simulink model "identification_sl"  (R2021b)
settings: Solver=FixedStepDiscrete  StartTime=0.0  StopTime=inf  FixedStep=0.5  RelTol=1e-3
undefined symbols (not defined in the file): arduino, fclose
libraries: sldrtlib x1
settings Model: Creator=IST  LastModifiedBy=IST

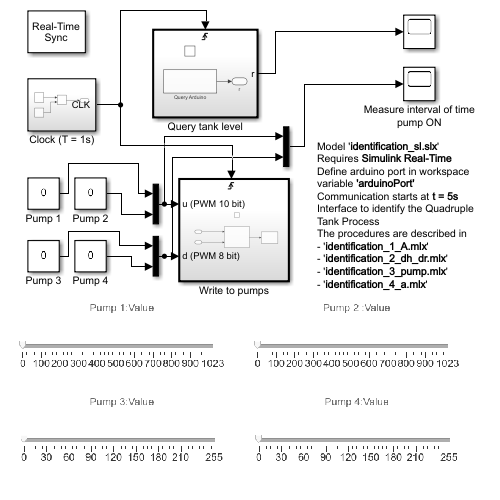
[thumbnail: Simulink's stored preview of the top-level diagram]
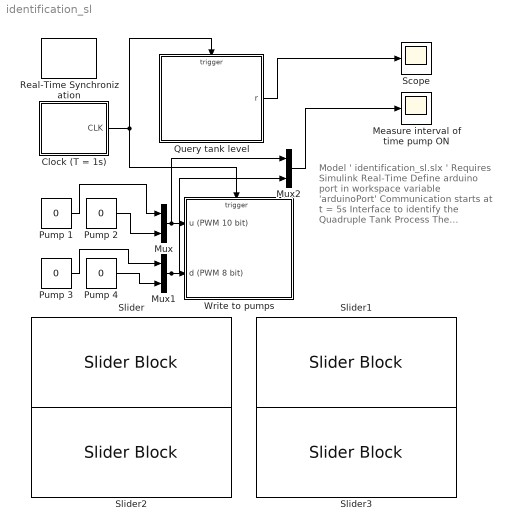
== system identification_sl ==
  note: Model ' identification_sl.slx '
      | Requires Simulink Real-Time
      | Define arduino port in workspace variable 'arduinoPort'
      | Communication starts at t = 5s
      | Interface to identify the Quadruple Tank Process
      | The procedures are described in
      | - ' identification_1_A.mlx '
      | - ' identification_2_dh_dr.mlx '
      | - ' identification_3_pump.mlx '
      | - ' identification_4_a.mlx '
  Clock (T = 1s) : Subsystem
  Measure interval of time pump ON : Scope
  Mux : Mux  Inputs=2
  Mux1 : Mux  Inputs=2
  Mux2 : Mux  Inputs=2
  Pump 1 : Constant  Value=0
  "Pump 2 " : Constant  Value=0
  Pump 3 : Constant  Value=0
  Pump 4 : Constant  Value=0
  Query tank level : Subsystem  Priority=1  InitFcn=|  StopFcn=fclose(arduino)
      | if exist('arduinoPort')
      | if ~isempty(instrfind)
      | fclose(instrfind);
      | delete(instrfind);
      | end
      | arduino = serial(arduinoPort,...
      |                 'BaudRate',9600,...
      |                 'ByteOrder','bigEndian',...
      |                 'DataBits',8,...
      |                 'StopBits',1,...
      |                 'Terminator','');
      | arduino.Parity = 'none';
      | fopen(arduino);
      | else
      | error("Error: Arduino port undefined. Define the port in workspace variable 'arduinoPort'.");
      | end
  Real-Time Synchronization : sldrtlib/Real-Time Synchronization  SampleTime=0.5  MaxMissedTicks=10  ShowMissedTicks=off  YieldWhenWaiting=off
  Scope : Scope
  Slider : SliderBlock  ScaleMax=1023
  Slider1 : SliderBlock  ScaleMax=1023
  Slider2 : SliderBlock  ScaleMax=255
  Slider3 : SliderBlock  ScaleMax=255
  Write to pumps : Subsystem  Priority=2
  wires:
  Mux1/1 -> Mux2/2, Write to pumps/2(d (PWM 8 bit))
  Query tank level/1(r) -> Scope/1
  Mux/1 -> Mux2/1, Write to pumps/1(u (PWM 10 bit))
  Pump 3/1 -> Mux1/1
  Pump 4/1 -> Mux1/2
  Clock (T = 1s)/1("CLK ") -> Write to pumps/Trigger, Query tank level/Trigger
  Pump 1/1 -> Mux/1
  "Pump 2 "/1 -> Mux/2
  Mux2/1 -> Measure interval of time pump ON/1

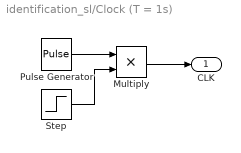
== system identification_sl/Clock (T = 1s) ==
  Multiply : Product
  Pulse Generator : DiscretePulseGenerator  PulseType=Time based  Period=1  PulseWidth=50
  Step : Step  Time=5  SampleTime=0
  "CLK " : Outport  VectorParamsAs1DForOutWhenUnconnected=off
  wires:
  Step/1 -> Multiply/2
  Pulse Generator/1 -> Multiply/1
  Multiply/1 -> "CLK "/1

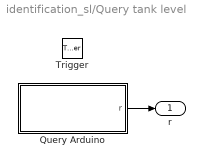
== system identification_sl/Query tank level ==
  Trigger : TriggerPort  VariantControl=Variant  PortDimensions=1
  Query Arduino : MATLAB Function  TreatAsAtomicUnit=on
  r : Outport  VectorParamsAs1DForOutWhenUnconnected=off
  wires:
  Query Arduino/1(r) -> r/1

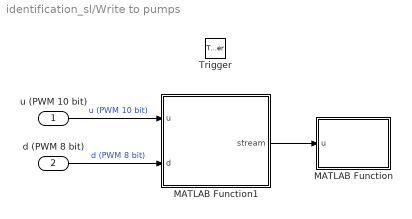
== system identification_sl/Write to pumps ==
  u (PWM 10 bit) : Inport
  d (PWM 8 bit) : Inport  Port=2
  Trigger : TriggerPort  VariantControl=Variant  PortDimensions=1
  MATLAB Function : MATLAB Function  TreatAsAtomicUnit=on
  MATLAB Function1 : MATLAB Function  TreatAsAtomicUnit=on
  wires:
  u (PWM 10 bit)/1 -> MATLAB Function1/1(u)  "u (PWM 10 bit)"
  d (PWM 8 bit)/1 -> MATLAB Function1/2(d)  "d (PWM 8 bit)"
  MATLAB Function1/1(stream) -> MATLAB Function/1(u)

== matlab function identification_sl/Write to pumps/MATLAB Function ==
  data: u input
function toArduino(u)
% Find arduino serial object
coder.extrinsic('instrfind'); 
persistent arduino;
if isempty(arduino)
    arduino = instrfind('Status','open','Baud',9600);
end
% Send metadata
fprintf(arduino, "#16");
% Send actuation inputs
fwrite(arduino,u,'uint16');
end

== matlab function identification_sl/Query tank level/Query Arduino ==
  data: r output
function r = queryArduino()
% Find arduino serial object
coder.extrinsic('instrfind'); 
persistent arduino;
if isempty(arduino)
    arduino = instrfind('Status','open','Baud',9600);
end

% Query arduino
fprintf(arduino, '$');
% Ignore metadata
fread(arduino,[4 1],'uint8');
% Read water-level data
aux = fread(arduino,[5 1],'uint16');
u = zeros(5,1);
u(5) = double(aux(5,1));
for i = 1:4
    u(i) = double(aux(i,1));
    u(i) = (u(5)-u(i))/u(i);
end
r = u(1:4);
end

== matlab function identification_sl/Write to pumps/MATLAB Function1 ==
  data: u input; stream output; d input
function stream = packPWM10bit(u,d)
    %% Saturation 
    u(u<0) = 0;
    u(u>2^10-1) =2^10-1;
    d(d<0) = 0;
    d(d>2^8-1) =2^8-1;
    %% Pack PWM 
    stream = uint16(zeros(3,1));
    % First two actuation pump signals of 10 bits are sent individually
    stream(1:2) = uint16(round(u)); 
    % Two disturbance pump signals of 8 bits are sent together as a 16 bit
    % uint16_t
    stream(3) = uint16(round(d(1))*2^8+round(d(2)));
end
